simulink model "Can_send_receive"  (R2024a)
settings: Solver=FixedStepAuto  StartTime=0.0  StopTime=20  RelTol=1e-3  EnableMultiTasking=on
undefined symbols (not defined in the file): CAN, FD
libraries: stmutilitieslib x68, simulink x36, stm32blockslib x17, canfdmsglib x10, stm32h7xxblockslib x3
(part 2 of 2)

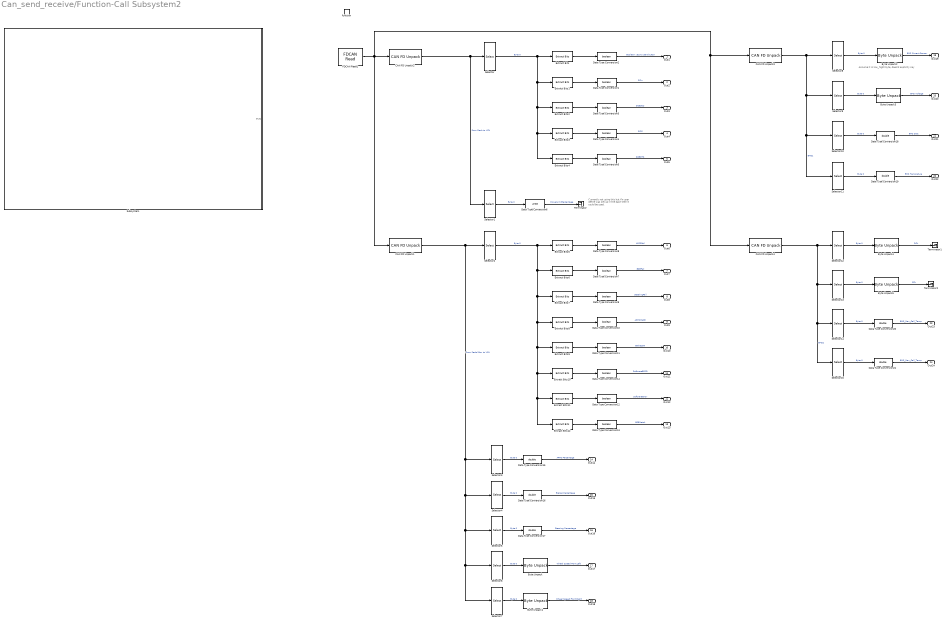
== system Can_send_receive/Function-Call Subsystem2 ==
  note: Assume it is low_hight byte, doesnt explicity say
  note: Currently not using this but if a user define was set up in the dash then it could be used.
  function : TriggerPort  TriggerType=function-call  VariantControl=(inherit)
  Byte Unpack{,1..5} (6 alike) : stmutilitieslib/Byte Unpack  dimensions={[1]}  datatypes={'uint16'}  byteAlign=1  blockPlatform=stm32f4discovery
  CAN FD Unpack1 : canfdmsglib/CAN FD Unpack  MsgList=(none)  MsgName=Msg  ProtocolMode=CAN  MsgIDType=Standard (11-bit identifier)  MsgIdentifier=1  MsgLength=8  SignalInfo={}  IDPort=off  TimestampPort=off  ErrorPort=off  RemotePort=off  LengthPort=off  StatusPort=off  BRSPort=off  ESIPort=off  DLCPort=off  ApplyMinMax=off
      settings: LibrarySourceBlock=stmutilitieslib/CAN FD Unpack  DataFormat=raw data
  CAN FD Unpack2 : canfdmsglib/CAN FD Unpack  MsgList=(none)  MsgName=Msg  ProtocolMode=CAN  MsgIDType=Standard (11-bit identifier)  MsgIdentifier=2  MsgLength=8  SignalInfo={}  IDPort=off  TimestampPort=off  ErrorPort=off  RemotePort=off  LengthPort=off  StatusPort=off  BRSPort=off  ESIPort=off  DLCPort=off  ApplyMinMax=off
      settings: LibrarySourceBlock=stmutilitieslib/CAN FD Unpack  DataFormat=raw data
  CAN FD Unpack3 : canfdmsglib/CAN FD Unpack  MsgList=(none)  MsgName=Msg  ProtocolMode=CAN  MsgIDType=Standard (11-bit identifier)  MsgIdentifier=4  MsgLength=8  SignalInfo={}  IDPort=off  TimestampPort=off  ErrorPort=off  RemotePort=off  LengthPort=off  StatusPort=off  BRSPort=off  ESIPort=off  DLCPort=off  ApplyMinMax=off
      settings: LibrarySourceBlock=stmutilitieslib/CAN FD Unpack  DataFormat=raw data
  CAN FD Unpack4 : canfdmsglib/CAN FD Unpack  MsgList=(none)  MsgName=Msg  ProtocolMode=CAN  MsgIDType=Standard (11-bit identifier)  MsgIdentifier=5  MsgLength=8  SignalInfo={}  IDPort=off  TimestampPort=off  ErrorPort=off  RemotePort=off  LengthPort=off  StatusPort=off  BRSPort=off  ESIPort=off  DLCPort=off  ApplyMinMax=off
      settings: LibrarySourceBlock=stmutilitieslib/CAN FD Unpack  DataFormat=raw data
  Data Type Conversion{1..5,7..14} (13 alike) : DataTypeConversion  OutDataTypeStr=boolean  SaturateOnIntegerOverflow=off  RndMeth=Floor
  Data Type Conversion{15..21} (7 alike) : DataTypeConversion  OutDataTypeStr=double  SaturateOnIntegerOverflow=off  RndMeth=Floor
  Data Type Conversion6 : DataTypeConversion  OutDataTypeStr=uint8  SaturateOnIntegerOverflow=off  RndMeth=Floor
  Extract Bits : simulink/Logic and Bit Operations/Extract Bits  bitsToExtract=Range of bits  numBits=8  bitIdxRange=[0]  outScalingMode=Treat bit field as an integer
  Extract Bits1 : simulink/Logic and Bit Operations/Extract Bits  bitsToExtract=Range of bits  numBits=8  bitIdxRange=[3]  outScalingMode=Treat bit field as an integer
  Extract Bits10 : simulink/Logic and Bit Operations/Extract Bits  bitsToExtract=Range of bits  numBits=8  bitIdxRange=[5]  outScalingMode=Treat bit field as an integer
  Extract Bits11 : simulink/Logic and Bit Operations/Extract Bits  bitsToExtract=Range of bits  numBits=8  bitIdxRange=[6]  outScalingMode=Treat bit field as an integer
  Extract Bits12 : simulink/Logic and Bit Operations/Extract Bits  bitsToExtract=Range of bits  numBits=8  bitIdxRange=[7]  outScalingMode=Treat bit field as an integer
  Extract Bits2 : simulink/Logic and Bit Operations/Extract Bits  bitsToExtract=Range of bits  numBits=8  bitIdxRange=[4]  outScalingMode=Treat bit field as an integer
  Extract Bits3 : simulink/Logic and Bit Operations/Extract Bits  bitsToExtract=Range of bits  numBits=8  bitIdxRange=[5]  outScalingMode=Treat bit field as an integer
  Extract Bits4 : simulink/Logic and Bit Operations/Extract Bits  bitsToExtract=Range of bits  numBits=8  bitIdxRange=[6]  outScalingMode=Treat bit field as an integer
  Extract Bits5 : simulink/Logic and Bit Operations/Extract Bits  bitsToExtract=Range of bits  numBits=8  bitIdxRange=[0]  outScalingMode=Treat bit field as an integer
  Extract Bits6 : simulink/Logic and Bit Operations/Extract Bits  bitsToExtract=Range of bits  numBits=8  bitIdxRange=[1]  outScalingMode=Treat bit field as an integer
  Extract Bits7 : simulink/Logic and Bit Operations/Extract Bits  bitsToExtract=Range of bits  numBits=8  bitIdxRange=[2]  outScalingMode=Treat bit field as an integer
  Extract Bits8 : simulink/Logic and Bit Operations/Extract Bits  bitsToExtract=Range of bits  numBits=8  bitIdxRange=[3]  outScalingMode=Treat bit field as an integer
  Extract Bits9 : simulink/Logic and Bit Operations/Extract Bits  bitsToExtract=Range of bits  numBits=8  bitIdxRange=[4]  outScalingMode=Treat bit field as an integer
  FDCAN Read1 : stm32blockslib/FDCAN Read  FDCANModule=FDCAN1  BlockMode=Receive  OperationReadMode=Data  OperationWriteMode=Data  ReadSource=FIFO 0  BufferNumber=0  OutputTypeReadMode=Packed  DataFormatWriteMode=Raw data  CANFrameType=CAN-FD  IdentifierTypeVia=Dialog  IdentifierType=Standard (11-bit identifier)  IdentifierVia=Inport  Identifier=100  DataLengthVia=Inport  DataLength=64  OutputIdType=off  IsBitRateSwitchingEnabled=off  TransmitRemoteFrame=off  OutputFrameType=off  OutputBRS=off  OutputRemoteFrame=off  OutputTxFifoLevel=off  OutputRxFifoLevel=off  OutputStatus=off  Timeout=0.001  SampleTime=-1
      settings: LibrarySourceBlock=stm32l5xxblockslib/FDCAN Read
  Selector : Selector  InputPortWidth=8  IndexOptions=Index vector (dialog)  Indices=[1 ]  OutputSizes=1
  Selector1 : Selector  InputPortWidth=8  IndexOptions=Index vector (dialog)  Indices=[2 ]  OutputSizes=1
  Selector{10..11,14..15} (4 alike) : Selector  InputPortWidth=8  IndexOptions=Index vector (dialog)  Indices=[5 ]  OutputSizes=1
  Selector12 : Selector  InputPortWidth=8  IndexOptions=Index vector (dialog)  Indices=[1 2 ]  OutputSizes=1
  Selector13 : Selector  InputPortWidth=8  IndexOptions=Index vector (dialog)  Indices=[3 4 ]  OutputSizes=1
  Selector2 : Selector  InputPortWidth=8  IndexOptions=Index vector (dialog)  Indices=[1 ]  OutputSizes=1
  Selector3 : Selector  InputPortWidth=8  IndexOptions=Index vector (dialog)  Indices=[2 ]  OutputSizes=1
  Selector4 : Selector  InputPortWidth=8  IndexOptions=Index vector (dialog)  Indices=[3 ]  OutputSizes=1
  Selector5 : Selector  InputPortWidth=8  IndexOptions=Index vector (dialog)  Indices=[4 ]  OutputSizes=1
  Selector6 : Selector  InputPortWidth=8  IndexOptions=Index vector (dialog)  Indices=[5 6 ]  OutputSizes=1
  Selector7 : Selector  InputPortWidth=8  IndexOptions=Index vector (dialog)  Indices=[7 8 ]  OutputSizes=1
  Selector8 : Selector  InputPortWidth=8  IndexOptions=Index vector (dialog)  Indices=[1 2 ]  OutputSizes=1
  Selector9 : Selector  InputPortWidth=8  IndexOptions=Index vector (dialog)  Indices=[3 4 ]  OutputSizes=1
  Subsystem : Subsystem
      mask Display: image('ALL Can.jpg');
  Terminator : Terminator
  Terminator1 : Terminator
  Terminator2 : Terminator
  Out1 : Outport
  Out2 : Outport  Port=2
  Out3 : Outport  Port=3
  Out4 : Outport  Port=4
  Out5 : Outport  Port=5
  Out6 : Outport  Port=6
  Out7 : Outport  Port=7
  Out8 : Outport  Port=8
  Out9 : Outport  Port=9
  Out10 : Outport  Port=10
  Out11 : Outport  Port=11
  Out12 : Outport  Port=12
  Out13 : Outport  Port=13
  Out14 : Outport  Port=14
  Out15 : Outport  Port=15
  Out16 : Outport  Port=16
  Out17 : Outport  Port=17
  Out18 : Outport  Port=18
  Out19 : Outport  Port=19
  Out20 : Outport  Port=20
  Out21 : Outport  Port=21
  Out22 : Outport  Port=22
  Out23 : Outport  Port=23
  Out24 : Outport  Port=24
  wires:
  CAN FD Unpack2/1 -> Selector1/1, Selector/1  "From Dash to VCU"
  FDCAN Read1/1 -> CAN FD Unpack1/1, CAN FD Unpack4/1, CAN FD Unpack3/1, CAN FD Unpack2/1
  Selector/1 -> Extract Bits4/1, Extract Bits3/1, Extract Bits2/1, Extract Bits1/1, Extract Bits/1  "Byte 0"
  Extract Bits/1 -> Data Type Conversion2/1
  Data Type Conversion2/1 -> Out1/1  "Boolean yes/no start button"
  Extract Bits1/1 -> Data Type Conversion1/1
  Data Type Conversion1/1 -> Out2/1  "SCin"
  Extract Bits2/1 -> Data Type Conversion3/1
  Data Type Conversion3/1 -> Out3/1  "SCEstop"
  Extract Bits3/1 -> Data Type Conversion4/1
  Data Type Conversion4/1 -> Out4/1  "SCIS"
  Extract Bits4/1 -> Data Type Conversion5/1
  Data Type Conversion5/1 -> Out5/1  "SCBOTS"
  Selector1/1 -> Data Type Conversion6/1  "Byte 0"
  Data Type Conversion6/1 -> Terminator/1  "PowerLimitPercentage"
  CAN FD Unpack1/1 -> Selector7/1, Selector6/1, Selector5/1, Selector4/1, Selector3/1, Selector2/1  "From Pedal Box to VCU"
  Data Type Conversion9/1 -> Out8/1  "SteeringFail"
  Extract Bits7/1 -> Data Type Conversion9/1
  Extract Bits6/1 -> Data Type Conversion7/1
  Extract Bits9/1 -> Data Type Conversion11/1
  Extract Bits5/1 -> Data Type Conversion8/1
  Extract Bits8/1 -> Data Type Conversion10/1
  Data Type Conversion7/1 -> Out7/1  "BSEFail"
  Data Type Conversion8/1 -> Out6/1  "APPSFail"
  Data Type Conversion10/1 -> Out9/1  "APPSMatch"
  Data Type Conversion11/1 -> Out10/1  "BrakesON"
  Extract Bits11/1 -> Data Type Conversion12/1
  Extract Bits12/1 -> Data Type Conversion13/1
  Data Type Conversion13/1 -> Out13/1  "BSEMatch"
  Selector2/1 -> Extract Bits12/1, Extract Bits11/1, Extract Bits10/1, Extract Bits9/1, Extract Bits8/1, Extract Bits7/1, Extract Bits6/1, Extract Bits5/1  "Byte 0"
  Data Type Conversion12/1 -> Out12/1  "SoftwareError"
  Data Type Conversion14/1 -> Out11/1  "SoftwareBSPD"
  Extract Bits10/1 -> Data Type Conversion14/1
  Selector3/1 -> Data Type Conversion15/1  "Byte 0"
  Data Type Conversion15/1 -> Out14/1  "APPS Percentage"
  Selector4/1 -> Data Type Conversion16/1  "Byte 0"
  Data Type Conversion16/1 -> Out15/1  "Brakes Percentage"
  Selector5/1 -> Data Type Conversion17/1  "Byte 0"
  Data Type Conversion17/1 -> Out16/1  "Steering Percentage"
  Selector6/1 -> Byte Unpack/1  "Byte 0"
  Byte Unpack/1 -> Out17/1  "Wheel Speed Front Left"
  Selector7/1 -> Byte Unpack1/1  "Byte 0"
  Byte Unpack1/1 -> Out18/1  "Wheel Speed Front Right"
  CAN FD Unpack3/1 -> Selector11/1, Selector10/1, Selector9/1, Selector8/1  "BMS1"
  Selector8/1 -> Byte Unpack2/1  "Byte 0"
  Byte Unpack2/1 -> Out19/1  "BMS Current Sensor"
  Selector9/1 -> Byte Unpack3/1  "Byte 0"
  Byte Unpack3/1 -> Out20/1  "BMS Voltage"
  Selector10/1 -> Data Type Conversion18/1  "Byte 0"
  Data Type Conversion18/1 -> Out21/1  "BMS SOC"
  Selector11/1 -> Data Type Conversion19/1  "Byte 0"
  Data Type Conversion19/1 -> Out22/1  "BMS Temprature"
  CAN FD Unpack4/1 -> Selector15/1, Selector14/1, Selector13/1, Selector12/1  "BMS2"
  Selector12/1 -> Byte Unpack4/1  "Byte 0"
  Byte Unpack4/1 -> Terminator1/1  "DCL"
  Selector13/1 -> Byte Unpack5/1  "Byte 0"
  Byte Unpack5/1 -> Terminator2/1  "CCL"
  Selector14/1 -> Data Type Conversion20/1  "Byte 0"
  Data Type Conversion20/1 -> Out23/1  "BMS_Max_Cell_Temp"
  Selector15/1 -> Data Type Conversion21/1  "Byte 0"
  Data Type Conversion21/1 -> Out24/1  "BMS_Max_Cell_Temp"

== system Can_send_receive/If Action Subsystem2 ==
  In1 : Inport
  Action Port : ActionPort  ActionPortLabel=case [ 138 ]:
  Out1 : Outport
  wires:
  In1/1 -> Out1/1

== system Can_send_receive/If Action Subsystem3 ==
  In1 : Inport
  Action Port : ActionPort  ActionPortLabel=case [ 95 ]:
  Out1 : Outport
  wires:
  In1/1 -> Out1/1

== system Can_send_receive/If Action Subsystem4 ==
  In1 : Inport
  Action Port : ActionPort  ActionPortLabel=case [ 73 ]:
  Out1 : Outport
  wires:
  In1/1 -> Out1/1

== system Can_send_receive/If Action Subsystem5 ==
  In1 : Inport
  Action Port : ActionPort  ActionPortLabel=case [ 168 ]:
  Out1 : Outport
  wires:
  In1/1 -> Out1/1

== system Can_send_receive/If Action Subsystem6 ==
  In1 : Inport
  Action Port : ActionPort  ActionPortLabel=case [ 74 ]:
  Out1 : Outport
  wires:
  In1/1 -> Out1/1

== system Can_send_receive/If Action Subsystem7 ==
  In1 : Inport
  Action Port : ActionPort  ActionPortLabel=case [ 235 ]:
  Out1 : Outport
  wires:
  In1/1 -> Out1/1

== system Can_send_receive/Subsystem ==
  Constant2 : Constant
  Out1 : Outport
  wires:
  Constant2/1 -> Out1/1

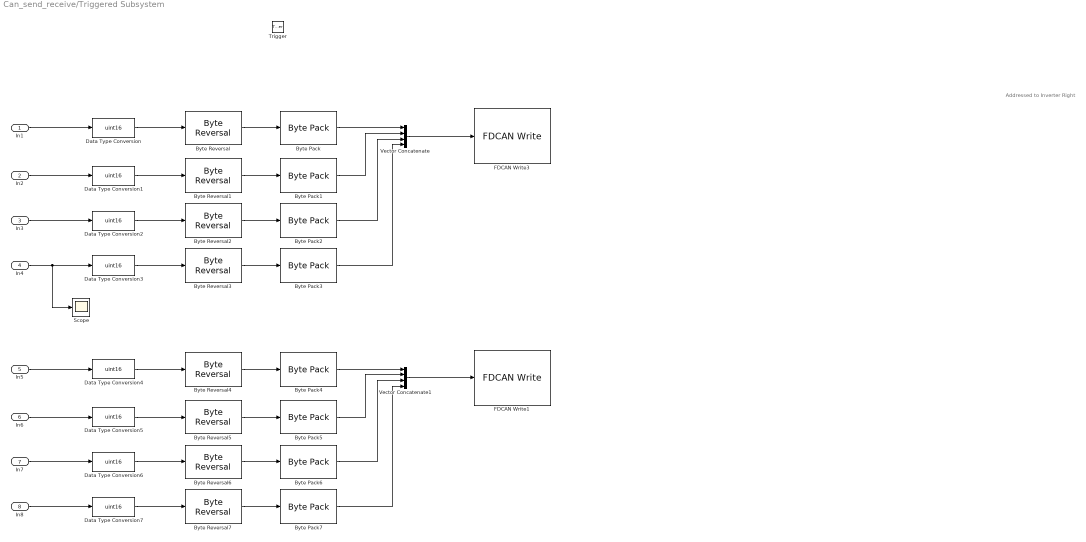
== system Can_send_receive/Triggered Subsystem ==
  note: Addressed to Inverter Right
  In1 : Inport
  In2 : Inport  Port=2
  In3 : Inport  Port=3
  In4 : Inport  Port=4
  In5 : Inport  Port=5
  In6 : Inport  Port=6
  In7 : Inport  Port=7
  In8 : Inport  Port=8
  Trigger : TriggerPort  TriggerType=function-call  VariantControl=(inherit)
  Byte Pack{,1..7} (8 alike) : stmutilitieslib/Byte Pack  datatypes={'uint16'}  byteAlign=1  blockPlatform=stm32f4discovery
  Byte Reversal{,1..7} (8 alike) : stmutilitieslib/Byte Reversal  numInp=1  blockPlatform=stm32f4discovery
  Data Type Conversion{,1..7} (8 alike) : DataTypeConversion  OutDataTypeStr=uint16  SaturateOnIntegerOverflow=off  RndMeth=Floor
  FDCAN Write1 : stm32blockslib/FDCAN Write  FDCANModule=FDCAN2  BlockMode=Transmit  OperationReadMode=Data  OperationWriteMode=Data  ReadSource=FIFO 0  BufferNumber=0  OutputTypeReadMode=Unpacked  DataFormatWriteMode=Raw data  CANFrameType=CAN  IdentifierTypeVia=Dialog  IdentifierType=Standard (11-bit identifier)  IdentifierVia=Dialog  Identifier=9  DataLengthVia=Dialog  DataLength=8  OutputIdType=off  IsBitRateSwitchingEnabled=off  TransmitRemoteFrame=off  OutputFrameType=off  OutputBRS=off  OutputRemoteFrame=off  OutputTxFifoLevel=off  OutputRxFifoLevel=off  OutputStatus=off  Timeout=1  SampleTime=-1
      settings: LibrarySourceBlock=stm32l5xxblockslib/FDCAN Write
  FDCAN Write3 : stm32blockslib/FDCAN Write  FDCANModule=FDCAN2  BlockMode=Transmit  OperationReadMode=Data  OperationWriteMode=Data  ReadSource=FIFO 0  BufferNumber=0  OutputTypeReadMode=Unpacked  DataFormatWriteMode=Raw data  CANFrameType=CAN  IdentifierTypeVia=Dialog  IdentifierType=Standard (11-bit identifier)  IdentifierVia=Dialog  Identifier=8  DataLengthVia=Dialog  DataLength=8  OutputIdType=off  IsBitRateSwitchingEnabled=off  TransmitRemoteFrame=off  OutputFrameType=off  OutputBRS=off  OutputRemoteFrame=off  OutputTxFifoLevel=off  OutputRxFifoLevel=off  OutputStatus=off  Timeout=1  SampleTime=-1
      settings: LibrarySourceBlock=stm32l5xxblockslib/FDCAN Write
  Scope : Scope
  Vector Concatenate : Concatenate  NumInputs=4
  Vector Concatenate1 : Concatenate  NumInputs=4
  wires:
  Byte Reversal/1 -> Byte Pack/1
  Byte Pack/1 -> Vector Concatenate/1
  Data Type Conversion/1 -> Byte Reversal/1
  In1/1 -> Data Type Conversion/1
  Byte Pack1/1 -> Vector Concatenate/2
  Byte Reversal1/1 -> Byte Pack1/1
  Data Type Conversion1/1 -> Byte Reversal1/1
  Byte Pack2/1 -> Vector Concatenate/3
  Byte Reversal2/1 -> Byte Pack2/1
  Data Type Conversion2/1 -> Byte Reversal2/1
  Byte Pack3/1 -> Vector Concatenate/4
  Byte Reversal3/1 -> Byte Pack3/1
  Data Type Conversion3/1 -> Byte Reversal3/1
  In2/1 -> Data Type Conversion1/1
  In3/1 -> Data Type Conversion2/1
  In4/1 -> Scope/1, Data Type Conversion3/1
  Vector Concatenate/1 -> FDCAN Write3/1
  Byte Pack6/1 -> Vector Concatenate1/3
  Byte Reversal7/1 -> Byte Pack7/1
  Vector Concatenate1/1 -> FDCAN Write1/1
  Byte Pack5/1 -> Vector Concatenate1/2
  Byte Pack7/1 -> Vector Concatenate1/4
  Byte Pack4/1 -> Vector Concatenate1/1
  Data Type Conversion7/1 -> Byte Reversal7/1
  Data Type Conversion4/1 -> Byte Reversal4/1
  Byte Reversal5/1 -> Byte Pack5/1
  Data Type Conversion5/1 -> Byte Reversal5/1
  Byte Reversal6/1 -> Byte Pack6/1
  Data Type Conversion6/1 -> Byte Reversal6/1
  Byte Reversal4/1 -> Byte Pack4/1
  In8/1 -> Data Type Conversion7/1
  In7/1 -> Data Type Conversion6/1
  In6/1 -> Data Type Conversion5/1
  In5/1 -> Data Type Conversion4/1

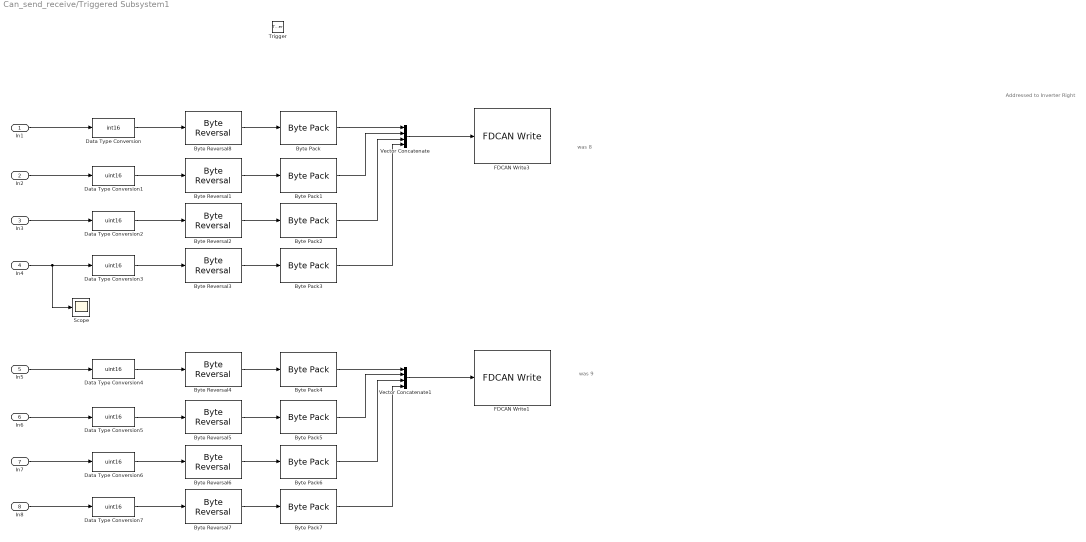
== system Can_send_receive/Triggered Subsystem1 ==
  note: was 9
  note: was 8
  note: Addressed to Inverter Right
  In1 : Inport
  In2 : Inport  Port=2
  In3 : Inport  Port=3
  In4 : Inport  Port=4
  In5 : Inport  Port=5
  In6 : Inport  Port=6
  In7 : Inport  Port=7
  In8 : Inport  Port=8
  Trigger : TriggerPort  TriggerType=function-call  VariantControl=(inherit)
  Byte Pack : stmutilitieslib/Byte Pack  datatypes={'int16'}  byteAlign=1  blockPlatform=stm32f4discovery
  Byte Pack{1..7} (7 alike) : stmutilitieslib/Byte Pack  datatypes={'uint16'}  byteAlign=1  blockPlatform=stm32f4discovery
  Byte Reversal{1..8} (8 alike) : stmutilitieslib/Byte Reversal  numInp=1  blockPlatform=stm32f4discovery
  Data Type Conversion : DataTypeConversion  OutDataTypeStr=int16  SaturateOnIntegerOverflow=off  RndMeth=Floor
  Data Type Conversion{1..7} (7 alike) : DataTypeConversion  OutDataTypeStr=uint16  SaturateOnIntegerOverflow=off  RndMeth=Floor
  FDCAN Write1 : stm32blockslib/FDCAN Write  FDCANModule=FDCAN2  BlockMode=Transmit  OperationReadMode=Data  OperationWriteMode=Data  ReadSource=FIFO 0  BufferNumber=0  OutputTypeReadMode=Unpacked  DataFormatWriteMode=Raw data  CANFrameType=CAN  IdentifierTypeVia=Dialog  IdentifierType=Standard (11-bit identifier)  IdentifierVia=Dialog  Identifier=404  DataLengthVia=Dialog  DataLength=8  OutputIdType=off  IsBitRateSwitchingEnabled=off  TransmitRemoteFrame=off  OutputFrameType=off  OutputBRS=off  OutputRemoteFrame=off  OutputTxFifoLevel=off  OutputRxFifoLevel=off  OutputStatus=off  Timeout=1  SampleTime=-1
      settings: LibrarySourceBlock=stm32l5xxblockslib/FDCAN Write
  FDCAN Write3 : stm32blockslib/FDCAN Write  FDCANModule=FDCAN2  BlockMode=Transmit  OperationReadMode=Data  OperationWriteMode=Data  ReadSource=FIFO 0  BufferNumber=0  OutputTypeReadMode=Unpacked  DataFormatWriteMode=Raw data  CANFrameType=CAN  IdentifierTypeVia=Dialog  IdentifierType=Standard (11-bit identifier)  IdentifierVia=Dialog  Identifier=403  DataLengthVia=Dialog  DataLength=8  OutputIdType=off  IsBitRateSwitchingEnabled=off  TransmitRemoteFrame=off  OutputFrameType=off  OutputBRS=off  OutputRemoteFrame=off  OutputTxFifoLevel=off  OutputRxFifoLevel=off  OutputStatus=off  Timeout=1  SampleTime=-1
      settings: LibrarySourceBlock=stm32l5xxblockslib/FDCAN Write
  Scope : Scope
  Vector Concatenate : Concatenate  NumInputs=4
  Vector Concatenate1 : Concatenate  NumInputs=4
  wires:
  Data Type Conversion/1 -> Byte Reversal8/1
  Byte Pack/1 -> Vector Concatenate/1
  In1/1 -> Data Type Conversion/1
  Byte Pack1/1 -> Vector Concatenate/2
  Byte Reversal1/1 -> Byte Pack1/1
  Data Type Conversion1/1 -> Byte Reversal1/1
  Byte Pack2/1 -> Vector Concatenate/3
  Byte Reversal2/1 -> Byte Pack2/1
  Data Type Conversion2/1 -> Byte Reversal2/1
  Byte Pack3/1 -> Vector Concatenate/4
  Byte Reversal3/1 -> Byte Pack3/1
  Data Type Conversion3/1 -> Byte Reversal3/1
  In2/1 -> Data Type Conversion1/1
  In3/1 -> Data Type Conversion2/1
  In4/1 -> Scope/1, Data Type Conversion3/1
  Vector Concatenate/1 -> FDCAN Write3/1
  Byte Pack6/1 -> Vector Concatenate1/3
  Byte Reversal7/1 -> Byte Pack7/1
  Vector Concatenate1/1 -> FDCAN Write1/1
  Byte Pack5/1 -> Vector Concatenate1/2
  Byte Pack7/1 -> Vector Concatenate1/4
  Byte Pack4/1 -> Vector Concatenate1/1
  Data Type Conversion7/1 -> Byte Reversal7/1
  Data Type Conversion4/1 -> Byte Reversal4/1
  Byte Reversal5/1 -> Byte Pack5/1
  Data Type Conversion5/1 -> Byte Reversal5/1
  Byte Reversal6/1 -> Byte Pack6/1
  Data Type Conversion6/1 -> Byte Reversal6/1
  Byte Reversal4/1 -> Byte Pack4/1
  In8/1 -> Data Type Conversion7/1
  In7/1 -> Data Type Conversion6/1
  In6/1 -> Data Type Conversion5/1
  In5/1 -> Data Type Conversion4/1
  Byte Reversal8/1 -> Byte Pack/1

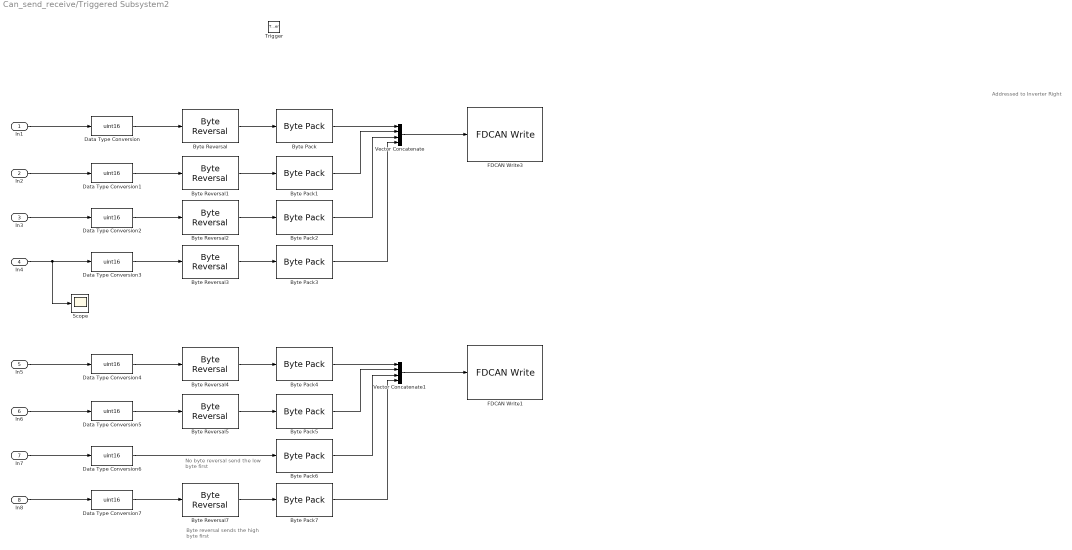
== system Can_send_receive/Triggered Subsystem2 ==
  note: Byte reversal sends the high byte first
  note: No byte reversal send the low byte first
  note: Addressed to Inverter Right
  In1 : Inport
  In2 : Inport  Port=2
  In3 : Inport  Port=3
  In4 : Inport  Port=4
  In5 : Inport  Port=5
  In6 : Inport  Port=6
  In7 : Inport  Port=7
  In8 : Inport  Port=8
  Trigger : TriggerPort  TriggerType=function-call  VariantControl=(inherit)
  Byte Pack{,1..7} (8 alike) : stmutilitieslib/Byte Pack  datatypes={'uint16'}  byteAlign=1  blockPlatform=stm32f4discovery
  Byte Reversal{,1..5,7} (7 alike) : stmutilitieslib/Byte Reversal  numInp=1  blockPlatform=stm32f4discovery
  Data Type Conversion{,1..7} (8 alike) : DataTypeConversion  OutDataTypeStr=uint16  SaturateOnIntegerOverflow=off  RndMeth=Floor
  FDCAN Write1 : stm32blockslib/FDCAN Write  FDCANModule=FDCAN2  BlockMode=Transmit  OperationReadMode=Data  OperationWriteMode=Data  ReadSource=FIFO 0  BufferNumber=0  OutputTypeReadMode=Unpacked  DataFormatWriteMode=Raw data  CANFrameType=CAN  IdentifierTypeVia=Dialog  IdentifierType=Standard (11-bit identifier)  IdentifierVia=Dialog  Identifier=9  DataLengthVia=Dialog  DataLength=8  OutputIdType=off  IsBitRateSwitchingEnabled=off  TransmitRemoteFrame=off  OutputFrameType=off  OutputBRS=off  OutputRemoteFrame=off  OutputTxFifoLevel=off  OutputRxFifoLevel=off  OutputStatus=off  Timeout=1  SampleTime=-1
      settings: LibrarySourceBlock=stm32l5xxblockslib/FDCAN Write
  FDCAN Write3 : stm32blockslib/FDCAN Write  FDCANModule=FDCAN2  BlockMode=Transmit  OperationReadMode=Data  OperationWriteMode=Data  ReadSource=FIFO 0  BufferNumber=0  OutputTypeReadMode=Unpacked  DataFormatWriteMode=Raw data  CANFrameType=CAN  IdentifierTypeVia=Dialog  IdentifierType=Standard (11-bit identifier)  IdentifierVia=Dialog  Identifier=8  DataLengthVia=Dialog  DataLength=8  OutputIdType=off  IsBitRateSwitchingEnabled=off  TransmitRemoteFrame=off  OutputFrameType=off  OutputBRS=off  OutputRemoteFrame=off  OutputTxFifoLevel=off  OutputRxFifoLevel=off  OutputStatus=off  Timeout=1  SampleTime=-1
      settings: LibrarySourceBlock=stm32l5xxblockslib/FDCAN Write
  Scope : Scope
  Vector Concatenate : Concatenate  NumInputs=4
  Vector Concatenate1 : Concatenate  NumInputs=4
  wires:
  Byte Reversal/1 -> Byte Pack/1
  Byte Pack/1 -> Vector Concatenate/1
  Data Type Conversion/1 -> Byte Reversal/1
  In1/1 -> Data Type Conversion/1
  Byte Pack1/1 -> Vector Concatenate/2
  Byte Reversal1/1 -> Byte Pack1/1
  Data Type Conversion1/1 -> Byte Reversal1/1
  Byte Pack2/1 -> Vector Concatenate/3
  Byte Reversal2/1 -> Byte Pack2/1
  Data Type Conversion2/1 -> Byte Reversal2/1
  Byte Pack3/1 -> Vector Concatenate/4
  Byte Reversal3/1 -> Byte Pack3/1
  Data Type Conversion3/1 -> Byte Reversal3/1
  In2/1 -> Data Type Conversion1/1
  In3/1 -> Data Type Conversion2/1
  In4/1 -> Scope/1, Data Type Conversion3/1
  Vector Concatenate/1 -> FDCAN Write3/1
  Byte Pack6/1 -> Vector Concatenate1/3
  Byte Reversal7/1 -> Byte Pack7/1
  Vector Concatenate1/1 -> FDCAN Write1/1
  Byte Pack5/1 -> Vector Concatenate1/2
  Byte Pack7/1 -> Vector Concatenate1/4
  Byte Pack4/1 -> Vector Concatenate1/1
  Data Type Conversion7/1 -> Byte Reversal7/1
  Data Type Conversion4/1 -> Byte Reversal4/1
  Byte Reversal5/1 -> Byte Pack5/1
  Data Type Conversion5/1 -> Byte Reversal5/1
  Data Type Conversion6/1 -> Byte Pack6/1
  Byte Reversal4/1 -> Byte Pack4/1
  In8/1 -> Data Type Conversion7/1
  In7/1 -> Data Type Conversion6/1
  In6/1 -> Data Type Conversion5/1
  In5/1 -> Data Type Conversion4/1

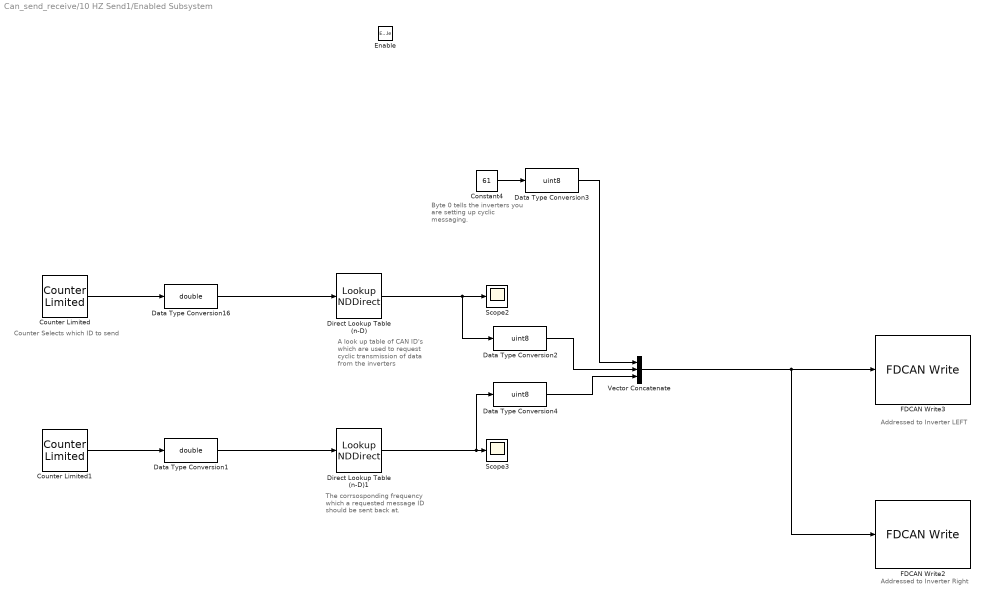
== system Can_send_receive/10 HZ Send1/Enabled Subsystem ==
  note: The corrsosponding frequency which a requested message ID should be sent back at.
  note: A look up table of CAN ID's which are used to request cyclic transmission of data from the inverters
  note: Byte 0 tells the inverters you are setting up cyclic messaging.
  note: Addressed to Inverter LEFT
  note: Counter Selects which ID to send
  note: Addressed to Inverter Right
  Enable : EnablePort
  Constant4 : Constant  Value=61
  Counter Limited : simulink/Sources/Counter Limited  uplimit=5  tsamp=-1
  Counter Limited1 : simulink/Sources/Counter Limited  uplimit=5  tsamp=-1
  Data Type Conversion1 : DataTypeConversion  OutDataTypeStr=double  SaturateOnIntegerOverflow=off  RndMeth=Floor
  Data Type Conversion16 : DataTypeConversion  OutDataTypeStr=double  SaturateOnIntegerOverflow=off  RndMeth=Floor
  Data Type Conversion2 : DataTypeConversion  OutDataTypeStr=uint8  SaturateOnIntegerOverflow=off  RndMeth=Floor
  Data Type Conversion3 : DataTypeConversion  OutDataTypeStr=uint8  SaturateOnIntegerOverflow=off  RndMeth=Floor
  Data Type Conversion4 : DataTypeConversion  OutDataTypeStr=uint8  SaturateOnIntegerOverflow=off  RndMeth=Floor
  Direct Lookup Table (n-D) : LookupNDDirect  NumberOfTableDimensions=1  Table=[235 74 168 73 95 138]
  Direct Lookup Table (n-D)1 : LookupNDDirect  NumberOfTableDimensions=1  Table=[235 74 168 73 95 138]
  FDCAN Write2 : stm32blockslib/FDCAN Write  FDCANModule=FDCAN2  BlockMode=Transmit  OperationReadMode=Data  OperationWriteMode=Data  ReadSource=FIFO 0  BufferNumber=0  OutputTypeReadMode=Unpacked  DataFormatWriteMode=Raw data  CANFrameType=CAN  IdentifierTypeVia=Dialog  IdentifierType=Standard (11-bit identifier)  IdentifierVia=Dialog  Identifier=529  DataLengthVia=Dialog  DataLength=3  OutputIdType=off  IsBitRateSwitchingEnabled=off  TransmitRemoteFrame=off  OutputFrameType=off  OutputBRS=off  OutputRemoteFrame=off  OutputTxFifoLevel=off  OutputRxFifoLevel=off  OutputStatus=off  Timeout=1  SampleTime=-1
      settings: LibrarySourceBlock=stm32l5xxblockslib/FDCAN Write
  FDCAN Write3 : stm32blockslib/FDCAN Write  FDCANModule=FDCAN2  BlockMode=Transmit  OperationReadMode=Data  OperationWriteMode=Data  ReadSource=FIFO 0  BufferNumber=0  OutputTypeReadMode=Unpacked  DataFormatWriteMode=Raw data  CANFrameType=CAN  IdentifierTypeVia=Dialog  IdentifierType=Standard (11-bit identifier)  IdentifierVia=Dialog  Identifier=528  DataLengthVia=Dialog  DataLength=3  OutputIdType=off  IsBitRateSwitchingEnabled=off  TransmitRemoteFrame=off  OutputFrameType=off  OutputBRS=off  OutputRemoteFrame=off  OutputTxFifoLevel=off  OutputRxFifoLevel=off  OutputStatus=off  Timeout=1  SampleTime=-1
      settings: LibrarySourceBlock=stm32l5xxblockslib/FDCAN Write
  Scope2 : Scope
  Scope3 : Scope
  Vector Concatenate : Concatenate  NumInputs=3
  wires:
  Direct Lookup Table (n-D)1/1 -> Data Type Conversion4/1, Scope3/1
  Data Type Conversion1/1 -> Direct Lookup Table (n-D)1/1
  Data Type Conversion16/1 -> Direct Lookup Table (n-D)/1
  Direct Lookup Table (n-D)/1 -> Data Type Conversion2/1, Scope2/1
  Counter Limited1/1 -> Data Type Conversion1/1
  Counter Limited/1 -> Data Type Conversion16/1
  Vector Concatenate/1 -> FDCAN Write2/1, FDCAN Write3/1
  Data Type Conversion3/1 -> Vector Concatenate/1
  Data Type Conversion4/1 -> Vector Concatenate/3
  Data Type Conversion2/1 -> Vector Concatenate/2
  Constant4/1 -> Data Type Conversion3/1

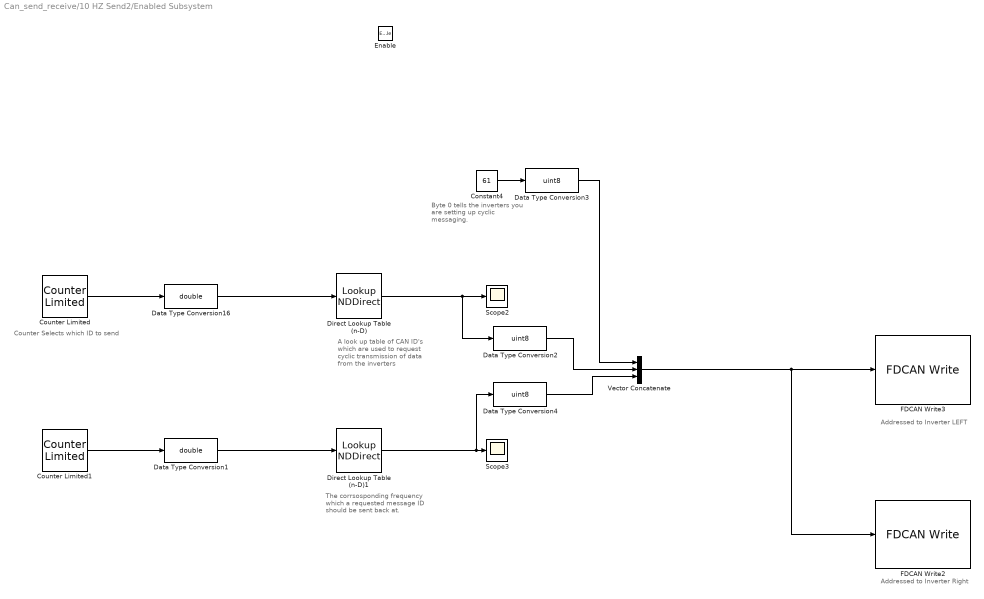
== system Can_send_receive/10 HZ Send2/Enabled Subsystem ==
  note: The corrsosponding frequency which a requested message ID should be sent back at.
  note: A look up table of CAN ID's which are used to request cyclic transmission of data from the inverters
  note: Byte 0 tells the inverters you are setting up cyclic messaging.
  note: Addressed to Inverter LEFT
  note: Counter Selects which ID to send
  note: Addressed to Inverter Right
  Enable : EnablePort
  Constant4 : Constant  Value=61
  Counter Limited : simulink/Sources/Counter Limited  uplimit=5  tsamp=-1
  Counter Limited1 : simulink/Sources/Counter Limited  uplimit=5  tsamp=-1
  Data Type Conversion1 : DataTypeConversion  OutDataTypeStr=double  SaturateOnIntegerOverflow=off  RndMeth=Floor
  Data Type Conversion16 : DataTypeConversion  OutDataTypeStr=double  SaturateOnIntegerOverflow=off  RndMeth=Floor
  Data Type Conversion2 : DataTypeConversion  OutDataTypeStr=uint8  SaturateOnIntegerOverflow=off  RndMeth=Floor
  Data Type Conversion3 : DataTypeConversion  OutDataTypeStr=uint8  SaturateOnIntegerOverflow=off  RndMeth=Floor
  Data Type Conversion4 : DataTypeConversion  OutDataTypeStr=uint8  SaturateOnIntegerOverflow=off  RndMeth=Floor
  Direct Lookup Table (n-D) : LookupNDDirect  NumberOfTableDimensions=1  Table=[235 74 168 73 95 138]
  Direct Lookup Table (n-D)1 : LookupNDDirect  NumberOfTableDimensions=1  Table=[235 74 168 73 95 138]
  FDCAN Write2 : stm32blockslib/FDCAN Write  FDCANModule=FDCAN2  BlockMode=Transmit  OperationReadMode=Data  OperationWriteMode=Data  ReadSource=FIFO 0  BufferNumber=0  OutputTypeReadMode=Unpacked  DataFormatWriteMode=Raw data  CANFrameType=CAN  IdentifierTypeVia=Dialog  IdentifierType=Standard (11-bit identifier)  IdentifierVia=Dialog  Identifier=529  DataLengthVia=Dialog  DataLength=3  OutputIdType=off  IsBitRateSwitchingEnabled=off  TransmitRemoteFrame=off  OutputFrameType=off  OutputBRS=off  OutputRemoteFrame=off  OutputTxFifoLevel=off  OutputRxFifoLevel=off  OutputStatus=off  Timeout=1  SampleTime=-1
      settings: LibrarySourceBlock=stm32l5xxblockslib/FDCAN Write
  FDCAN Write3 : stm32blockslib/FDCAN Write  FDCANModule=FDCAN2  BlockMode=Transmit  OperationReadMode=Data  OperationWriteMode=Data  ReadSource=FIFO 0  BufferNumber=0  OutputTypeReadMode=Unpacked  DataFormatWriteMode=Raw data  CANFrameType=CAN  IdentifierTypeVia=Dialog  IdentifierType=Standard (11-bit identifier)  IdentifierVia=Dialog  Identifier=528  DataLengthVia=Dialog  DataLength=3  OutputIdType=off  IsBitRateSwitchingEnabled=off  TransmitRemoteFrame=off  OutputFrameType=off  OutputBRS=off  OutputRemoteFrame=off  OutputTxFifoLevel=off  OutputRxFifoLevel=off  OutputStatus=off  Timeout=1  SampleTime=-1
      settings: LibrarySourceBlock=stm32l5xxblockslib/FDCAN Write
  Scope2 : Scope
  Scope3 : Scope
  Vector Concatenate : Concatenate  NumInputs=3
  wires:
  Direct Lookup Table (n-D)1/1 -> Data Type Conversion4/1, Scope3/1
  Data Type Conversion1/1 -> Direct Lookup Table (n-D)1/1
  Data Type Conversion16/1 -> Direct Lookup Table (n-D)/1
  Direct Lookup Table (n-D)/1 -> Data Type Conversion2/1, Scope2/1
  Counter Limited1/1 -> Data Type Conversion1/1
  Counter Limited/1 -> Data Type Conversion16/1
  Vector Concatenate/1 -> FDCAN Write2/1, FDCAN Write3/1
  Data Type Conversion3/1 -> Vector Concatenate/1
  Data Type Conversion4/1 -> Vector Concatenate/3
  Data Type Conversion2/1 -> Vector Concatenate/2
  Constant4/1 -> Data Type Conversion3/1

== system Can_send_receive/Function-Call Subsystem/If Action Subsystem1 ==
  In1 : Inport
  Action Port : ActionPort  ActionPortLabel=case [ 138 ]:
  Out1 : Outport
  wires:
  In1/1 -> Out1/1

== system Can_send_receive/Function-Call Subsystem/If Action Subsystem10 ==
  In1 : Inport
  Action Port : ActionPort  ActionPortLabel=case [ 168 ]:
  Out1 : Outport
  wires:
  In1/1 -> Out1/1

== system Can_send_receive/Function-Call Subsystem/If Action Subsystem11 ==
  In1 : Inport
  Action Port : ActionPort  ActionPortLabel=case [ 74 ]:
  Out1 : Outport
  wires:
  In1/1 -> Out1/1

== system Can_send_receive/Function-Call Subsystem/If Action Subsystem12 ==
  In1 : Inport
  Action Port : ActionPort  ActionPortLabel=case [ 235 ]:
  Out1 : Outport
  wires:
  In1/1 -> Out1/1

== system Can_send_receive/Function-Call Subsystem/If Action Subsystem2 ==
  In1 : Inport
  Action Port : ActionPort  ActionPortLabel=case [ 95 ]:
  Out1 : Outport
  wires:
  In1/1 -> Out1/1

== system Can_send_receive/Function-Call Subsystem/If Action Subsystem3 ==
  In1 : Inport
  Action Port : ActionPort  ActionPortLabel=case [ 73 ]:
  Out1 : Outport
  wires:
  In1/1 -> Out1/1

== system Can_send_receive/Function-Call Subsystem/If Action Subsystem4 ==
  In1 : Inport
  Action Port : ActionPort  ActionPortLabel=case [ 168 ]:
  Out1 : Outport
  wires:
  In1/1 -> Out1/1

== system Can_send_receive/Function-Call Subsystem/If Action Subsystem5 ==
  In1 : Inport
  Action Port : ActionPort  ActionPortLabel=case [ 74 ]:
  Out1 : Outport
  wires:
  In1/1 -> Out1/1

== system Can_send_receive/Function-Call Subsystem/If Action Subsystem6 ==
  In1 : Inport
  Action Port : ActionPort  ActionPortLabel=case [ 235 ]:
  Out1 : Outport
  wires:
  In1/1 -> Out1/1

== system Can_send_receive/Function-Call Subsystem/If Action Subsystem7 ==
  In1 : Inport
  Action Port : ActionPort  ActionPortLabel=case [ 138 ]:
  Out1 : Outport
  wires:
  In1/1 -> Out1/1

== system Can_send_receive/Function-Call Subsystem/If Action Subsystem8 ==
  In1 : Inport
  Action Port : ActionPort  ActionPortLabel=case [ 95 ]:
  Out1 : Outport
  wires:
  In1/1 -> Out1/1

== system Can_send_receive/Function-Call Subsystem/If Action Subsystem9 ==
  In1 : Inport
  Action Port : ActionPort  ActionPortLabel=case [ 73 ]:
  Out1 : Outport
  wires:
  In1/1 -> Out1/1

== system Can_send_receive/Function-Call Subsystem1/Subsystem ==
  Constant2 : Constant
  Out1 : Outport
  wires:
  Constant2/1 -> Out1/1

== system Can_send_receive/Function-Call Subsystem2/Subsystem ==
  Constant2 : Constant
  Out1 : Outport
  wires:
  Constant2/1 -> Out1/1
